simulink model "Assign_Task5and6"  (R2023a)
settings: Solver=ode1  StartTime=0.0  StopTime=30  FixedStep=Ts  MaxStep=Ts  RelTol=1e-3
model workspace (MAT data in the model file):
  wsw = 2000
values from neighbouring files (symbols this model uses):
  fg = 50    [Parameters.m]
  Rtpu = Xtpu/40    (= 0.00375)    [Parameters.m]
  S0non = 1000e6    (= 1000000000)    [Parameters.m]
  Svsc = 100e6    (= 100000000)    [Parameters.m]
  tonvsc = 1e-3    (= 0.001)    [Parameters.m]
  Ts = 20e-6    (= 2e-05)    [Parameters.m]
  Vhv = 22e3    (= 22000)    [Parameters.m]
  Vmv = 22e3    (= 22000)    [Parameters.m]
  wc1 = wsw1/10    (= 848.230016469)    [Parameters.m]
  wpq1 = wc1/10    (= 84.8230016469)    [Parameters.m]
  wsw1 = ksw1*2*pi*fg    (= 8482.30016469)    [Parameters.m]
  Xtpu = 0.15    [Parameters.m]
undefined symbols (not defined in the file or in its folder): D11, Delta, Kf, r, tfilt, theta0
libraries: simulink_extras x20, spsGroundLib x18, spsCurrentMeasurementLib x12, spsVoltageMeasurementLib x12, pid_lib x7, slpidlib x7, spsThreePhaseParallelRLCLoadLib x6, spsControlledVoltageSourceLib x6, powerlib_meascontrol x5, spsThreePhaseBreakerLib x4, eeTransforms x4, spsabctoAlphaBetaZeroLib x3
(part 3 of 3)

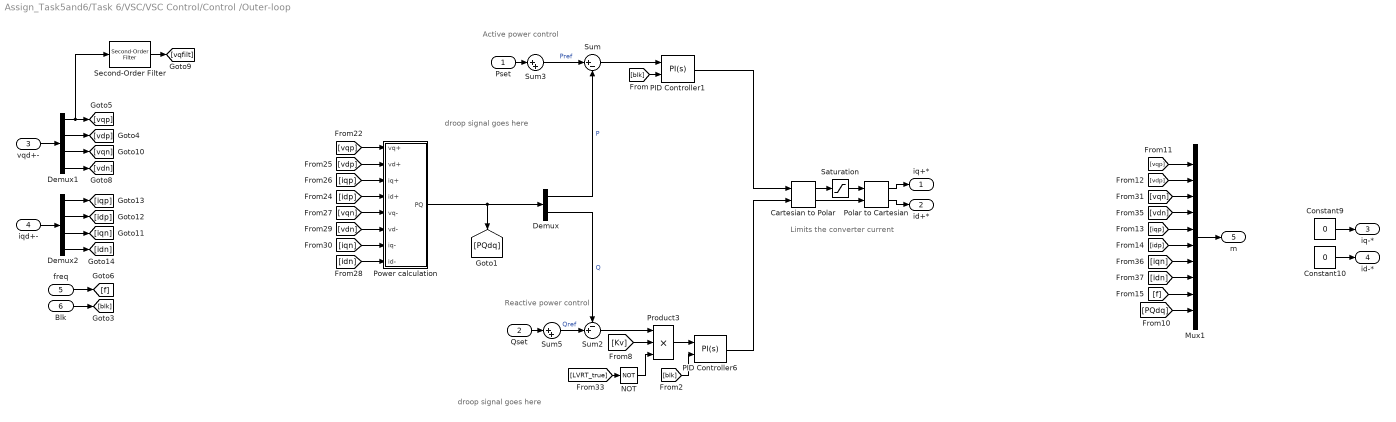
== system Assign_Task5and6/Task 6/VSC/VSC Control/Control /Outer-loop ==
  note: droop signal goes here
  note: Limits the converter current
  note: Reactive power control
  note: Active power control
  note: droop signal goes here
  Pset : Inport
  Qset : Inport  Port=2
  vqd+- : Inport  Port=3
  iqd+- : Inport  Port=4
  freq : Inport  Port=5
  Blk : Inport  Port=6
  Cartesian to Polar : simulink_extras/Transformations/Cartesian to Polar
  Constant10 : Constant  Value=0
  Constant9 : Constant  Value=0
  Demux : Demux  Outputs=2
  Demux1 : Demux
  Demux2 : Demux
  Mux1 : Mux  Inputs=10
  NOT : Logic  Operator=NOT  IconShape=distinctive  AllPortsSameDT=off  OutDataTypeStr=boolean
  PID Controller1 : slpidlib/PID Controller  Controller=PI  Form=Ideal  TimeDomain=Continuous-time  UseExternalTs=off  SampleTime=-1  IntegratorMethod=Forward Euler  FilterMethod=Forward Euler  ControllerParametersSource=internal  P=kp_pq  I=1/ti_pq  UseKiTs=off  D=0  N=100  UseFilter=on  TunerSelectOption=Transfer Function Based (PID Tuner App)  InitialConditionSource=internal  InitialConditionForIntegrator=0  InitialConditionForFilter=0  DifferentiatorICPrevScaledInput=0  ExternalReset=level  TrackingMode=off  Kt=1  LimitOutput=off  SatLimitsSource=internal  UpperSaturationLimit=inf  LowerSaturationLimit=-inf  LinearizeAsGain=on  AntiWindupMode=none  Kb=1  LimitIntegrator=off  UpperIntegratorSaturationLimit=inf  LowerIntegratorSaturationLimit=-inf  POutMin=[]  POutMax=[]  IOutMin=[]  IOutMax=[]  DOutMin=[]  DOutMax=[]  NOutMin=[]  NOutMax=[]  SumOutMin=[]  SumOutMax=[]  SaturationOutMin=[]  SaturationOutMax=[]  PParamMin=[]  PParamMax=[]  IParamMin=[]  IParamMax=[]  DParamMin=[]  DParamMax=[]  NParamMin=[]  NParamMax=[]  KbParamMin=[]  KbParamMax=[]  KtParamMin=[]  KtParamMax=[]  KbOutMin=[]  KbOutMax=[]  KtOutMin=[]  KtOutMax=[]  IntegratorOutMin=[]  IntegratorOutMax=[]  FilterOutMin=[]  FilterOutMax=[]  SumI1OutMin=[]  SumI1OutMax=[]  SumI2OutMin=[]  SumI2OutMax=[]  SumI3OutMin=[]  SumI3OutMax=[]  SumI4OutMin=[]  SumI4OutMax=[]  SumDOutMin=[]  SumDOutMax=[]  DifferentiatorOutMin=[]  DifferentiatorOutMax=[]  FilterDiffOutCoefMin=[]  FilterDiffOutCoefMax=[]  ReciprocalOutMin=[]  ReciprocalOutMax=[]  SumDenOutMin=[]  SumDenOutMax=[]  SumNumOutMin=[]  SumNumOutMax=[]  DivideOutMin=[]  DivideOutMax=[]  UdiffTsProdOutMin=[]  UdiffTsProdOutMax=[]  NTsProdOutMin=[]  NTsProdOutMax=[]  UintegralTsProdOutMin=[]  UintegralTsProdOutMax=[]  UngainTsProdOutMin=[]  UngainTsProdOutMax=[]  ClampingZeroOutDataTypeStr=Inherit: Inherit via back propagation  ClampingZeroOutMin=[]  ClampingZeroOutMax=[]  FilterDenConstantOutDataTypeStr=Inherit: Inherit via back propagation  FilterDenConstantOutMin=[]  FilterDenConstantOutMax=[]  PCopyOutDataTypeStr=Inherit: Inherit via back propagation  PCopyOutMin=[]  PCopyOutMax=[]  NCopyOutDataTypeStr=Inherit: Inherit via back propagation  NCopyOutMin=[]  NCopyOutMax=[]  IntegratorContinuousStateAttributes=''  IntegratorStateMustResolveToSignalObject=off  IntegratorRTWStateStorageClass=Auto  FilterContinuousStateAttributes=''  FilterStateMustResolveToSignalObject=off  FilterRTWStateStorageClass=Auto  ParallelPVariant=Passthrough  IdealPVariant=InternalParameters  IVariant=InternalParameters  DVariant=Disabled  IntegratorVariant=Continuous  SatVariant=Disabled  AWVariant=Passthrough  PCopyVariant=Disabled  TRVariant=Disabled  FdbkBlocksVariant=Forward  IdealPFdbkVariant=Disabled  SatFdbkVariant=Disabled  DerivativeFilterVariant=Disabled  NVariant=Disabled  NCopyVariant=Disabled_SignalSpec  FilterICVariant=Disabled  IntegratorICVariant=InternalICs  ExternalResetVariant=ExternalReset  TRSumVariant=Passthrough  SumFdbkVariant=Disabled  SumVariant=Sum_PI  TsampFilterVariant=InternalTs  TsampNgainVariant=Passthrough  TsampIntegralVariant=Disabled_SignalSpec  ExternalSaturationOutDataTypeStr=Inherit: Same as second input
  PID Controller6 : slpidlib/PID Controller  Controller=PI  Form=Ideal  TimeDomain=Continuous-time  UseExternalTs=off  SampleTime=-1  IntegratorMethod=Forward Euler  FilterMethod=Forward Euler  ControllerParametersSource=internal  P=kp_pq  I=1/ti_pq  UseKiTs=off  D=0  N=100  UseFilter=on  TunerSelectOption=Transfer Function Based (PID Tuner App)  InitialConditionSource=internal  InitialConditionForIntegrator=0  InitialConditionForFilter=0  DifferentiatorICPrevScaledInput=0  ExternalReset=level  TrackingMode=off  Kt=1  LimitOutput=off  SatLimitsSource=internal  UpperSaturationLimit=inf  LowerSaturationLimit=-inf  LinearizeAsGain=on  AntiWindupMode=none  Kb=1  LimitIntegrator=off  UpperIntegratorSaturationLimit=inf  LowerIntegratorSaturationLimit=-inf  POutMin=[]  POutMax=[]  IOutMin=[]  IOutMax=[]  DOutMin=[]  DOutMax=[]  NOutMin=[]  NOutMax=[]  SumOutMin=[]  SumOutMax=[]  SaturationOutMin=[]  SaturationOutMax=[]  PParamMin=[]  PParamMax=[]  IParamMin=[]  IParamMax=[]  DParamMin=[]  DParamMax=[]  NParamMin=[]  NParamMax=[]  KbParamMin=[]  KbParamMax=[]  KtParamMin=[]  KtParamMax=[]  KbOutMin=[]  KbOutMax=[]  KtOutMin=[]  KtOutMax=[]  IntegratorOutMin=[]  IntegratorOutMax=[]  FilterOutMin=[]  FilterOutMax=[]  SumI1OutMin=[]  SumI1OutMax=[]  SumI2OutMin=[]  SumI2OutMax=[]  SumI3OutMin=[]  SumI3OutMax=[]  SumI4OutMin=[]  SumI4OutMax=[]  SumDOutMin=[]  SumDOutMax=[]  DifferentiatorOutMin=[]  DifferentiatorOutMax=[]  FilterDiffOutCoefMin=[]  FilterDiffOutCoefMax=[]  ReciprocalOutMin=[]  ReciprocalOutMax=[]  SumDenOutMin=[]  SumDenOutMax=[]  SumNumOutMin=[]  SumNumOutMax=[]  DivideOutMin=[]  DivideOutMax=[]  UdiffTsProdOutMin=[]  UdiffTsProdOutMax=[]  NTsProdOutMin=[]  NTsProdOutMax=[]  UintegralTsProdOutMin=[]  UintegralTsProdOutMax=[]  UngainTsProdOutMin=[]  UngainTsProdOutMax=[]  ClampingZeroOutDataTypeStr=Inherit: Inherit via back propagation  ClampingZeroOutMin=[]  ClampingZeroOutMax=[]  FilterDenConstantOutDataTypeStr=Inherit: Inherit via back propagation  FilterDenConstantOutMin=[]  FilterDenConstantOutMax=[]  PCopyOutDataTypeStr=Inherit: Inherit via back propagation  PCopyOutMin=[]  PCopyOutMax=[]  NCopyOutDataTypeStr=Inherit: Inherit via back propagation  NCopyOutMin=[]  NCopyOutMax=[]  IntegratorContinuousStateAttributes=''  IntegratorStateMustResolveToSignalObject=off  IntegratorRTWStateStorageClass=Auto  FilterContinuousStateAttributes=''  FilterStateMustResolveToSignalObject=off  FilterRTWStateStorageClass=Auto  ParallelPVariant=Passthrough  IdealPVariant=InternalParameters  IVariant=InternalParameters  DVariant=Disabled  IntegratorVariant=Continuous  SatVariant=Disabled  AWVariant=Passthrough  PCopyVariant=Disabled  TRVariant=Disabled  FdbkBlocksVariant=Forward  IdealPFdbkVariant=Disabled  SatFdbkVariant=Disabled  DerivativeFilterVariant=Disabled  NVariant=Disabled  NCopyVariant=Disabled_SignalSpec  FilterICVariant=Disabled  IntegratorICVariant=InternalICs  ExternalResetVariant=ExternalReset  TRSumVariant=Passthrough  SumFdbkVariant=Disabled  SumVariant=Sum_PI  TsampFilterVariant=InternalTs  TsampNgainVariant=Passthrough  TsampIntegralVariant=Disabled_SignalSpec  ExternalSaturationOutDataTypeStr=Inherit: Same as second input
  Polar to Cartesian : simulink_extras/Transformations/Polar to Cartesian
  Power calculation : Subsystem
  Product3 : Product  Inputs=3
  Saturation : Saturate  UpperLimit=Imax  LowerLimit=0
  Second-Order Filter : eeGeneralControl/Second-Order Filter  FilterType=Low-pass  fn=150  Zeta=0.9  Ts=-1  A0=0  Ph0=0  f0=0  b0=0
  Sum : Sum  Inputs=|+-
  Sum2 : Sum  Inputs=-+|
  Sum3 : Sum  Inputs=|++
  Sum5 : Sum  Inputs=|++
  iq+* : Outport
  id+* : Outport  Port=2
  iq-* : Outport  Port=3
  id-* : Outport  Port=4
  m : Outport  Port=5
  wires:
  Constant10/1 -> id-*/1
  Constant9/1 -> iq-*/1
  Qset/1 -> Sum5/1
  Cartesian to Polar/2 -> Polar to Cartesian/2
  Polar to Cartesian/1 -> iq+*/1
  Polar to Cartesian/2 -> id+*/1
  Cartesian to Polar/1 -> Saturation/1
  Saturation/1 -> Polar to Cartesian/1
  Demux/1 -> Sum/2  "P"
  Demux/2 -> Sum2/1  "Q"
  Sum3/1 -> Sum/1  "Pref"
  Sum5/1 -> Sum2/2  "Qref"
  [Kv] -> Product3/2
  Sum2/1 -> Product3/1
  Pset/1 -> Sum3/1
  PID Controller1/1 -> Cartesian to Polar/1
  Blk/1 -> [blk]
  freq/1 -> [f]
  [vqp] -> Mux1/1
  Mux1/1 -> m/1
  Product3/1 -> PID Controller6/1
  Sum/1 -> PID Controller1/1
  Second-Order Filter/1 -> [vqfilt]
  vqd+-/1 -> Demux1/1
  iqd+-/1 -> Demux2/1
  Demux1/1 -> Second-Order Filter/1, [vqp]
  Demux1/2 -> [vdp]
  Demux1/3 -> [vqn]
  Demux1/4 -> [vdn]
  Demux2/1 -> [iqp]
  Demux2/2 -> [idp]
  Demux2/3 -> [iqn]
  Demux2/4 -> [idn]
  [vqp] -> Power calculation/1(vq+)
  [iqp] -> Power calculation/3(iq+)
  Power calculation/1(PQ) -> [PQdq], Demux/1
  [idp] -> Power calculation/4(id+)
  [vdp] -> Power calculation/2(vd+)
  [vqn] -> Power calculation/5(vq-)
  [vdn] -> Power calculation/6(vd-)
  [iqn] -> Power calculation/7(iq-)
  [idn] -> Power calculation/8(id-)
  [LVRT_true] -> NOT/1
  NOT/1 -> Product3/3
  PID Controller6/1 -> Cartesian to Polar/2
  [vdp] -> Mux1/2
  [vqn] -> Mux1/3
  [vdn] -> Mux1/4
  [iqn] -> Mux1/7
  [idn] -> Mux1/8
  [f] -> Mux1/9
  [PQdq] -> Mux1/10
  [idp] -> Mux1/6
  [iqp] -> Mux1/5
  [blk] -> PID Controller1/2
  [blk] -> PID Controller6/2
  ? -> Sum5/2
  ? -> Sum3/2

== system Assign_Task5and6/Task 6/VSC/VSC Control/Measurement and PLL/PLL aligned with positive-sequence ==
  note: PLL
      | aligned with vd+
  Vabc : Inport
  0-vd=-vd : Gain  Gain=-1
  Clock : Clock  Commented=on
  Constant : Constant  Commented=on  Value=2*pi*fg
  Constant1 : Constant  Commented=on  Value=2*pi
  Constant2 : Constant  Commented=on  Value=2*pi
  Filter : Constant  Commented=on  Value=-tfilt*fg*2*pi
  Gain : Gain  Gain=1/(2*pi)
  Integrator : Integrator
  Mod : Math  Commented=on  Operator=mod
  Mod1 : Math  Commented=on  Operator=mod
  Notch filter : Subsystem  Commented=through
  PID Controller : slpidlib/PID Controller  Commented=on  Controller=PI  Form=Ideal  TimeDomain=Continuous-time  UseExternalTs=off  SampleTime=-1  IntegratorMethod=Forward Euler  FilterMethod=Forward Euler  ControllerParametersSource=internal  P=kp_pll  I=1/tau_pll  UseKiTs=off  D=0  N=100  UseFilter=on  TunerSelectOption=Transfer Function Based (PID Tuner App)  InitialConditionSource=internal  InitialConditionForIntegrator=2*pi*fg  InitialConditionForFilter=0  DifferentiatorICPrevScaledInput=0  ExternalReset=none  TrackingMode=off  Kt=1  LimitOutput=off  SatLimitsSource=internal  UpperSaturationLimit=1.1*2*pi*fg  LowerSaturationLimit=0.9*2*pi*fg  LinearizeAsGain=on  AntiWindupMode=clamping  Kb=1/kp_pll  LimitIntegrator=off  UpperIntegratorSaturationLimit=inf  LowerIntegratorSaturationLimit=-inf  POutMin=[]  POutMax=[]  IOutMin=[]  IOutMax=[]  DOutMin=[]  DOutMax=[]  NOutMin=[]  NOutMax=[]  SumOutMin=[]  SumOutMax=[]  SaturationOutMin=[]  SaturationOutMax=[]  PParamMin=[]  PParamMax=[]  IParamMin=[]  IParamMax=[]  DParamMin=[]  DParamMax=[]  NParamMin=[]  NParamMax=[]  KbParamMin=[]  KbParamMax=[]  KtParamMin=[]  KtParamMax=[]  KbOutMin=[]  KbOutMax=[]  KtOutMin=[]  KtOutMax=[]  IntegratorOutMin=[]  IntegratorOutMax=[]  FilterOutMin=[]  FilterOutMax=[]  SumI1OutMin=[]  SumI1OutMax=[]  SumI2OutMin=[]  SumI2OutMax=[]  SumI3OutMin=[]  SumI3OutMax=[]  SumI4OutMin=[]  SumI4OutMax=[]  SumDOutMin=[]  SumDOutMax=[]  DifferentiatorOutMin=[]  DifferentiatorOutMax=[]  FilterDiffOutCoefMin=[]  FilterDiffOutCoefMax=[]  ReciprocalOutMin=[]  ReciprocalOutMax=[]  SumDenOutMin=[]  SumDenOutMax=[]  SumNumOutMin=[]  SumNumOutMax=[]  DivideOutMin=[]  DivideOutMax=[]  UdiffTsProdOutMin=[]  UdiffTsProdOutMax=[]  NTsProdOutMin=[]  NTsProdOutMax=[]  UintegralTsProdOutMin=[]  UintegralTsProdOutMax=[]  UngainTsProdOutMin=[]  UngainTsProdOutMax=[]  ClampingZeroOutDataTypeStr=Inherit: Inherit via back propagation  ClampingZeroOutMin=[]  ClampingZeroOutMax=[]  FilterDenConstantOutDataTypeStr=Inherit: Inherit via back propagation  FilterDenConstantOutMin=[]  FilterDenConstantOutMax=[]  PCopyOutDataTypeStr=Inherit: Inherit via back propagation  PCopyOutMin=[]  PCopyOutMax=[]  NCopyOutDataTypeStr=Inherit: Inherit via back propagation  NCopyOutMin=[]  NCopyOutMax=[]  IntegratorContinuousStateAttributes=''  IntegratorStateMustResolveToSignalObject=off  IntegratorRTWStateStorageClass=Auto  FilterContinuousStateAttributes=''  FilterStateMustResolveToSignalObject=off  FilterRTWStateStorageClass=Auto  ParallelPVariant=Passthrough  IdealPVariant=InternalParameters  IVariant=InternalParameters  DVariant=Disabled  IntegratorVariant=Continuous  SatVariant=Disabled  AWVariant=Passthrough  PCopyVariant=Disabled  TRVariant=Disabled  FdbkBlocksVariant=Forward  IdealPFdbkVariant=Disabled  SatFdbkVariant=Disabled  DerivativeFilterVariant=Disabled  NVariant=Disabled  NCopyVariant=Disabled_SignalSpec  FilterICVariant=Disabled  IntegratorICVariant=InternalICs  ExternalResetVariant=Disabled  TRSumVariant=Passthrough  SumFdbkVariant=Disabled  SumVariant=Sum_PI  TsampFilterVariant=InternalTs  TsampNgainVariant=Passthrough  TsampIntegralVariant=Disabled_SignalSpec  ExternalSaturationOutDataTypeStr=Inherit: Same as second input
  Park transform : Subsystem  Commented=on
  Phase-sequence separation : Subsystem
  Subsystem : Subsystem
      mask Display: disp('PI\n')
  Switch : Switch  Commented=on  Criteria=u2 > Threshold  Threshold=0.3  SaturateOnIntegerOverflow=off  InputSameDT=off
  Terminator : Terminator
  Terminator1 : Terminator
  Terminator2 : Terminator
  Transformer Y/D1 : Constant  Commented=on  Value=-pi/6
  theta : Outport
  f : Outport  Port=2
  wires:
  Integrator/1 -> theta/1, Phase-sequence separation/2(Theta)
  Constant2/1 -> Mod1/1
  Constant1/1 -> Mod/2
  Gain/1 -> f/1
  0-vd=-vd/1 -> Subsystem/1(in)
  Clock/1 -> Switch/2
  Constant/1 -> Switch/1
  Subsystem/1(w) -> Gain/1, Integrator/1
  Vabc/1 -> Phase-sequence separation/1(abc)
  Phase-sequence separation/1(q+) -> Terminator/1
  Phase-sequence separation/2(d+) -> 0-vd=-vd/1  "vd+"
  Phase-sequence separation/3(q-) -> Terminator1/1
  Phase-sequence separation/4(d-) -> Terminator2/1

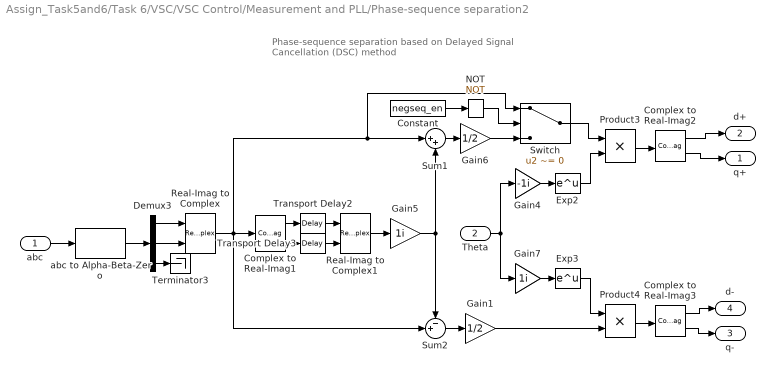
== system Assign_Task5and6/Task 6/VSC/VSC Control/Measurement and PLL/Phase-sequence separation2 ==
  note: Phase-sequence separation based on
      | Delayed Signal Cancellation (DSC) method
  abc : Inport
  Theta : Inport  Port=2
  Complex to Real-Imag1 : ComplexToRealImag
  Complex to Real-Imag2 : ComplexToRealImag
  Complex to Real-Imag3 : ComplexToRealImag
  Constant : Constant  Value=negseq_en
  Demux3 : Demux  Outputs=3
  Exp2 : Math  OutputSignalType=complex
  Exp3 : Math  OutputSignalType=complex
  Gain1 : Gain  Gain=1/2
  Gain4 : Gain  Gain=-1i
  Gain5 : Gain  Gain=1i
  Gain6 : Gain  Gain=1/2
  Gain7 : Gain  Gain=1i
  NOT : Logic  Operator=NOT  IconShape=distinctive  AllPortsSameDT=off  OutDataTypeStr=boolean
  Product3 : Product
  Product4 : Product
  Real-Imag to Complex : RealImagToComplex
  Real-Imag to Complex1 : RealImagToComplex
  Sum1 : Sum  Inputs=|++
  Sum2 : Sum  Inputs=-+|
  Switch : Switch  Criteria=u2 ~= 0  SaturateOnIntegerOverflow=off  InputSameDT=off
  Terminator3 : Terminator
  Transport Delay2 : TransportDelay  DelayTime=1/4*(1/50)
  Transport Delay3 : TransportDelay  DelayTime=1/4*(1/50)
  abc to Alpha-Beta-Zero : spsabctoAlphaBetaZeroLib/abc to Alpha-Beta-Zero
  q+ : Outport
  d+ : Outport  Port=2
  q- : Outport  Port=3
  d- : Outport  Port=4
  wires:
  NOT/1 -> Switch/2
  Constant/1 -> NOT/1
  Switch/1 -> Product3/1
  Gain6/1 -> Switch/3
  Sum2/1 -> Gain1/1
  Transport Delay2/1 -> Real-Imag to Complex1/1
  Demux3/1 -> Real-Imag to Complex/1
  Complex to Real-Imag1/2 -> Transport Delay3/1
  Gain1/1 -> Product4/2
  Real-Imag to Complex/1 -> Complex to Real-Imag1/1, Sum2/2, Sum1/1, Switch/1
  Complex to Real-Imag3/1 -> d-/1
  Real-Imag to Complex1/1 -> Gain5/1
  Complex to Real-Imag1/1 -> Transport Delay2/1
  Transport Delay3/1 -> Real-Imag to Complex1/2
  Demux3/2 -> Real-Imag to Complex/2
  Product3/1 -> Complex to Real-Imag2/1
  Product4/1 -> Complex to Real-Imag3/1
  abc to Alpha-Beta-Zero/1 -> Demux3/1
  abc/1 -> abc to Alpha-Beta-Zero/1
  Exp3/1 -> Product4/1
  Complex to Real-Imag3/2 -> q-/1
  Complex to Real-Imag2/2 -> q+/1
  Demux3/3 -> Terminator3/1
  Sum1/1 -> Gain6/1
  Gain5/1 -> Sum2/1, Sum1/2
  Exp2/1 -> Product3/2
  Gain4/1 -> Exp2/1
  Theta/1 -> Gain4/1, Gain7/1
  Gain7/1 -> Exp3/1
  Complex to Real-Imag2/1 -> d+/1

== system Assign_Task5and6/Task 6/VSC/VSC Control/Measurement and PLL/Phase-sequence separation3 ==
  note: Phase-sequence separation based on
      | Delayed Signal Cancellation (DSC) method
  abc : Inport
  Theta : Inport  Port=2
  Complex to Real-Imag1 : ComplexToRealImag
  Complex to Real-Imag2 : ComplexToRealImag
  Complex to Real-Imag3 : ComplexToRealImag
  Constant : Constant  Value=negseq_en
  Demux3 : Demux  Outputs=3
  Exp2 : Math  OutputSignalType=complex
  Exp3 : Math  OutputSignalType=complex
  Gain1 : Gain  Gain=1/2
  Gain4 : Gain  Gain=-1i
  Gain5 : Gain  Gain=1i
  Gain6 : Gain  Gain=1/2
  Gain7 : Gain  Gain=1i
  NOT : Logic  Operator=NOT  IconShape=distinctive  AllPortsSameDT=off  OutDataTypeStr=boolean
  Product3 : Product
  Product4 : Product
  Real-Imag to Complex : RealImagToComplex
  Real-Imag to Complex1 : RealImagToComplex
  Sum1 : Sum  Inputs=|++
  Sum2 : Sum  Inputs=-+|
  Switch : Switch  Criteria=u2 ~= 0  SaturateOnIntegerOverflow=off  InputSameDT=off
  Terminator3 : Terminator
  Transport Delay2 : TransportDelay  DelayTime=1/4*(1/50)
  Transport Delay3 : TransportDelay  DelayTime=1/4*(1/50)
  abc to Alpha-Beta-Zero : spsabctoAlphaBetaZeroLib/abc to Alpha-Beta-Zero
  q+ : Outport
  d+ : Outport  Port=2
  q- : Outport  Port=3
  d- : Outport  Port=4
  wires:
  Complex to Real-Imag2/1 -> d+/1
  Gain7/1 -> Exp3/1
  Theta/1 -> Gain7/1, Gain4/1
  Gain4/1 -> Exp2/1
  Exp2/1 -> Product3/2
  Gain5/1 -> Sum1/2, Sum2/1
  Sum1/1 -> Gain6/1
  Demux3/3 -> Terminator3/1
  Complex to Real-Imag2/2 -> q+/1
  Complex to Real-Imag3/2 -> q-/1
  Exp3/1 -> Product4/1
  abc/1 -> abc to Alpha-Beta-Zero/1
  abc to Alpha-Beta-Zero/1 -> Demux3/1
  Product4/1 -> Complex to Real-Imag3/1
  Product3/1 -> Complex to Real-Imag2/1
  Demux3/2 -> Real-Imag to Complex/2
  Transport Delay3/1 -> Real-Imag to Complex1/2
  Complex to Real-Imag1/1 -> Transport Delay2/1
  Real-Imag to Complex1/1 -> Gain5/1
  Complex to Real-Imag3/1 -> d-/1
  Real-Imag to Complex/1 -> Switch/1, Sum1/1, Sum2/2, Complex to Real-Imag1/1
  Gain1/1 -> Product4/2
  Complex to Real-Imag1/2 -> Transport Delay3/1
  Demux3/1 -> Real-Imag to Complex/1
  Transport Delay2/1 -> Real-Imag to Complex1/1
  Sum2/1 -> Gain1/1
  Gain6/1 -> Switch/3
  Switch/1 -> Product3/1
  Constant/1 -> NOT/1
  NOT/1 -> Switch/2

== system Assign_Task5and6/Task 6/VSC/VSC Control/Modulation/Corrects delay ==
  Clock : Clock
  Filter delay : Constant  Commented=on  Value=tfilt
  Gain : Gain  Gain=2*pi*fg
  Memory : Memory
  Sum : Sum  Inputs=|+-
  Sum1 : Sum  Inputs=|++
  Sum2 : Sum  Inputs=|++
  Transformer connection : Constant  Value=pi/6
  dphi : Outport
  wires:
  Clock/1 -> Memory/1, Sum/1
  Memory/1 -> Sum/2
  Sum1/1 -> Gain/1  "Td"
  Sum/1 -> Sum1/1  "Ts"
  Filter delay/1 -> Sum1/2  "Tf"
  Gain/1 -> Sum2/1
  Sum2/1 -> dphi/1
  Transformer connection/1 -> Sum2/2  "Tf"

== system Assign_Task5and6/Task 6/VSC/VSC Control/Modulation/Corrects delay1 ==
  Clock : Clock
  Filter delay : Constant  Commented=on  Value=tfilt
  Gain : Gain  Gain=-2*pi*fg
  Gain1 : Gain
  Memory : Memory
  Sum : Sum  Inputs=|+-
  Sum1 : Sum  Inputs=|++
  Sum2 : Sum  Inputs=|++
  Transformer connection : Constant  Value=pi/6
  dphi : Outport
  wires:
  Clock/1 -> Memory/1, Sum/1
  Memory/1 -> Sum/2
  Sum1/1 -> Gain/1  "Td"
  Sum/1 -> Sum1/1  "Ts"
  Filter delay/1 -> Sum1/2  "Tf"
  Gain/1 -> Sum2/1
  Sum2/1 -> Gain1/1
  Transformer connection/1 -> Sum2/2  "Tf"
  Gain1/1 -> dphi/1

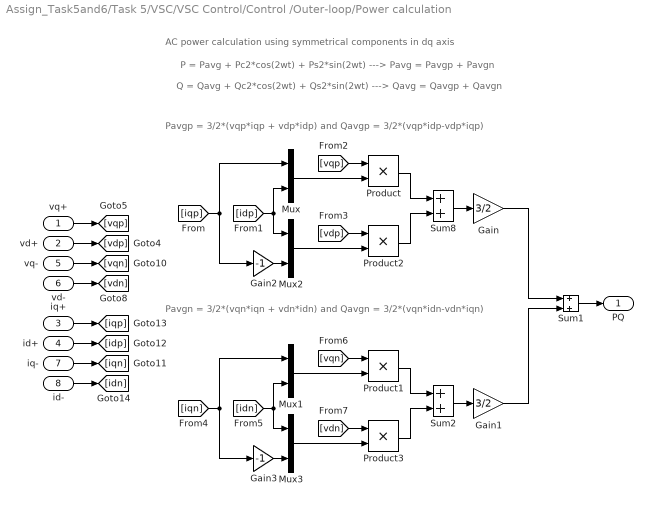
== system Assign_Task5and6/Task 5/VSC/VSC Control/Control /Outer-loop/Power calculation ==
  note: AC power calculation using symmetrical components in dq axis
  note: Pavgp = 3/2*(vqp*iqp + vdp*idp) and Qavgp = 3/2*(vqp*idp-vdp*iqp)
  note: P = Pavg + Pc2*cos(2wt) + Ps2*sin(2wt) ---> Pavg = Pavgp + Pavgn
  note: Q = Qavg + Qc2*cos(2wt) + Qs2*sin(2wt) ---> Qavg = Qavgp + Qavgn
  note: Pavgn = 3/2*(vqn*iqn + vdn*idn) and Qavgn = 3/2*(vqn*idn-vdn*iqn)
  vq+ : Inport
  vd+ : Inport  Port=2
  iq+ : Inport  Port=3
  id+ : Inport  Port=4
  vq- : Inport  Port=5
  vd- : Inport  Port=6
  iq- : Inport  Port=7
  id- : Inport  Port=8
  Gain : Gain  Gain=3/2
  Gain1 : Gain  Gain=3/2
  Gain2 : Gain  Gain=-1
  Gain3 : Gain  Gain=-1
  Mux{,1..3} (4 alike) : Mux  Inputs=2
  Product{,1..3} (4 alike) : Product
  Sum1 : Sum
  Sum2 : Sum
  Sum8 : Sum
  PQ : Outport
  wires:
  Sum8/1 -> Gain/1
  Gain2/1 -> Mux2/2
  Mux2/1 -> Product2/2
  Product2/1 -> Sum8/2
  Mux/1 -> Product/2
  Product/1 -> Sum8/1
  iq+/1 -> [iqp]
  [iqp] -> Gain2/1, Mux/1
  id+/1 -> [idp]
  [idp] -> Mux2/1, Mux/2
  vq+/1 -> [vqp]
  [vqp] -> Product/1
  vd+/1 -> [vdp]
  [vdp] -> Product2/1
  Gain/1 -> Sum1/1
  Sum1/1 -> PQ/1
  Gain3/1 -> Mux3/2
  Mux1/1 -> Product1/2
  Product3/1 -> Sum2/2
  Product1/1 -> Sum2/1
  [vdn] -> Product3/1
  Mux3/1 -> Product3/2
  [vqn] -> Product1/1
  Sum2/1 -> Gain1/1
  [iqn] -> Gain3/1, Mux1/1
  [idn] -> Mux3/1, Mux1/2
  vq-/1 -> [vqn]
  vd-/1 -> [vdn]
  iq-/1 -> [iqn]
  id-/1 -> [idn]
  Gain1/1 -> Sum1/2

== system Assign_Task5and6/Task 5/VSC/VSC Control/Measurement and PLL/PLL aligned with positive-sequence/Notch filter ==
  In : Inport
  Discrete Transfer Fcn : DiscreteTransferFcn  Numerator=[1, -2*cos(theta0), 1]  Denominator="[1, -2*cos(theta0)*r,  r^2]"
  Gain7 : Gain  Gain=Kf
  Out : Outport
  wires:
  Gain7/1 -> Discrete Transfer Fcn/1
  Discrete Transfer Fcn/1 -> Out/1
  In/1 -> Gain7/1

== system Assign_Task5and6/Task 5/VSC/VSC Control/Measurement and PLL/PLL aligned with positive-sequence/Park transform ==
  note: Park transform (q axis leading)
  abc : Inport
  theta : Inport  Port=2
  0 : Fcn  Expr=1/3*(u(1) + u(2) + u(3))
  Mux2 : Mux  Inputs=2
  Mux3 : Mux  Inputs=3
  d : Fcn  Expr=2/3*(u(1)*sin(u(4)) + u(2)*sin(u(4) - (2*pi)/3) + u(3)*sin(u(4) + (2*pi)/3))
  q : Fcn  Expr=2/3*(u(1)*cos(u(4)) + u(2)*cos(u(4) - (2*pi)/3) + u(3)*cos(u(4) + (2*pi)/3))
  qd0 : Outport  VectorParamsAs1DForOutWhenUnconnected=off
  wires:
  q/1 -> Mux3/1
  Mux2/1 -> q/1, 0/1, d/1
  0/1 -> Mux3/3
  d/1 -> Mux3/2
  theta/1 -> Mux2/2
  abc/1 -> Mux2/1
  Mux3/1 -> qd0/1

== system Assign_Task5and6/Task 5/VSC/VSC Control/Measurement and PLL/PLL aligned with positive-sequence/Phase-sequence separation ==
  note: Phase-sequence separation based on
      | Delayed Signal Cancellation (DSC) method
  abc : Inport
  Theta : Inport  Port=2
  Complex to Real-Imag1 : ComplexToRealImag
  Complex to Real-Imag2 : ComplexToRealImag
  Complex to Real-Imag3 : ComplexToRealImag
  Constant : Constant  Value=negseq_en
  Demux3 : Demux  Outputs=3
  Exp2 : Math  OutputSignalType=complex
  Exp3 : Math  OutputSignalType=complex
  Gain1 : Gain  Gain=1/2
  Gain4 : Gain  Gain=-1i
  Gain5 : Gain  Gain=1i
  Gain6 : Gain  Gain=1/2
  Gain7 : Gain  Gain=1i
  NOT : Logic  Operator=NOT  IconShape=distinctive  AllPortsSameDT=off  OutDataTypeStr=boolean
  Product3 : Product
  Product4 : Product
  Real-Imag to Complex : RealImagToComplex
  Real-Imag to Complex1 : RealImagToComplex
  Sum1 : Sum  Inputs=|++
  Sum2 : Sum  Inputs=-+|
  Switch : Switch  Criteria=u2 ~= 0  SaturateOnIntegerOverflow=off  InputSameDT=off
  Terminator3 : Terminator
  Transport Delay2 : TransportDelay  DelayTime=1/4*(1/50)
  Transport Delay3 : TransportDelay  DelayTime=1/4*(1/50)
  abc to Alpha-Beta-Zero : powerlib_meascontrol/Transformations/abc to Alpha-Beta-Zero
  q+ : Outport
  d+ : Outport  Port=2
  q- : Outport  Port=3
  d- : Outport  Port=4
  wires:
  NOT/1 -> Switch/2
  Constant/1 -> NOT/1
  Switch/1 -> Product3/1
  Gain6/1 -> Switch/3
  Sum2/1 -> Gain1/1
  Transport Delay2/1 -> Real-Imag to Complex1/1
  Demux3/1 -> Real-Imag to Complex/1
  Complex to Real-Imag1/2 -> Transport Delay3/1
  Gain1/1 -> Product4/2
  Real-Imag to Complex/1 -> Complex to Real-Imag1/1, Sum2/2, Sum1/1, Switch/1
  Complex to Real-Imag3/1 -> d-/1
  Real-Imag to Complex1/1 -> Gain5/1
  Complex to Real-Imag1/1 -> Transport Delay2/1
  Transport Delay3/1 -> Real-Imag to Complex1/2
  Demux3/2 -> Real-Imag to Complex/2
  Product3/1 -> Complex to Real-Imag2/1
  Product4/1 -> Complex to Real-Imag3/1
  abc to Alpha-Beta-Zero/1 -> Demux3/1
  abc/1 -> abc to Alpha-Beta-Zero/1
  Exp3/1 -> Product4/1
  Complex to Real-Imag3/2 -> q-/1
  Complex to Real-Imag2/2 -> q+/1
  Demux3/3 -> Terminator3/1
  Sum1/1 -> Gain6/1
  Gain5/1 -> Sum2/1, Sum1/2
  Exp2/1 -> Product3/2
  Gain4/1 -> Exp2/1
  Theta/1 -> Gain4/1, Gain7/1
  Gain7/1 -> Exp3/1
  Complex to Real-Imag2/1 -> d+/1

== system Assign_Task5and6/Task 5/VSC/VSC Control/Measurement and PLL/PLL aligned with positive-sequence/Subsystem ==
  note: PI controller with reset port and initial conditions restored after reset or after maximum/minimum values are reached
  in : Inport
  Reset : Inport  Port=2
  Compare To Constant2 : simulink/Logic and Bit Operations/Compare To Constant  relop=~=  const=0  OutDataTypeStr=boolean
  Constant2 : Constant  Value=2*pi*fg
  Gain : Gain  Gain=kp_pll
  Gain1 : Gain  Gain=kp_pll/tau_pll
  Integrator Limited : Integrator  ExternalReset=level  InitialCondition=2*pi*fg  UpperSaturationLimit=10.1*2*pi*fg  LowerSaturationLimit=0.09*2*pi*fg  ShowSaturationPort=on
  Memory1 : Memory
  NOT : Logic  Operator=NOT  IconShape=distinctive  AllPortsSameDT=off  OutDataTypeStr=boolean
  OR2 : Logic  Operator=OR  IconShape=distinctive  AllPortsSameDT=off  OutDataTypeStr=boolean
  Product : Product
  Sum : Sum
  Switch1 : Switch  SaturateOnIntegerOverflow=off  InputSameDT=off
  w : Outport
  wires:
  Switch1/1 -> w/1
  Product/1 -> Gain1/1, Gain/1
  Gain1/1 -> Integrator Limited/1
  Integrator Limited/2 -> Compare To Constant2/1, Switch1/2
  Compare To Constant2/1 -> Memory1/1
  OR2/1 -> Integrator Limited/2, NOT/1
  Constant2/1 -> Switch1/3
  Memory1/1 -> OR2/1
  Reset/1 -> OR2/2
  Gain/1 -> Sum/1
  Integrator Limited/1 -> Sum/2
  Sum/1 -> Switch1/1
  in/1 -> Product/1
  NOT/1 -> Product/2

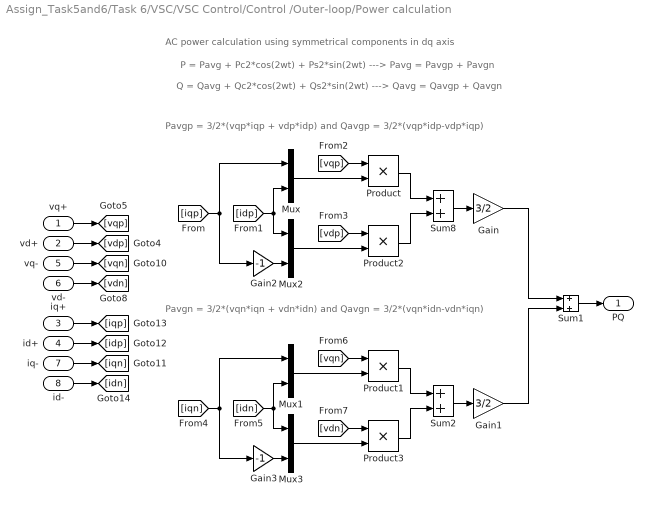
== system Assign_Task5and6/Task 6/VSC/VSC Control/Control /Outer-loop/Power calculation ==
  note: AC power calculation using symmetrical components in dq axis
  note: Pavgp = 3/2*(vqp*iqp + vdp*idp) and Qavgp = 3/2*(vqp*idp-vdp*iqp)
  note: P = Pavg + Pc2*cos(2wt) + Ps2*sin(2wt) ---> Pavg = Pavgp + Pavgn
  note: Q = Qavg + Qc2*cos(2wt) + Qs2*sin(2wt) ---> Qavg = Qavgp + Qavgn
  note: Pavgn = 3/2*(vqn*iqn + vdn*idn) and Qavgn = 3/2*(vqn*idn-vdn*iqn)
  vq+ : Inport
  vd+ : Inport  Port=2
  iq+ : Inport  Port=3
  id+ : Inport  Port=4
  vq- : Inport  Port=5
  vd- : Inport  Port=6
  iq- : Inport  Port=7
  id- : Inport  Port=8
  Gain : Gain  Gain=3/2
  Gain1 : Gain  Gain=3/2
  Gain2 : Gain  Gain=-1
  Gain3 : Gain  Gain=-1
  Mux{,1..3} (4 alike) : Mux  Inputs=2
  Product{,1..3} (4 alike) : Product
  Sum1 : Sum
  Sum2 : Sum
  Sum8 : Sum
  PQ : Outport
  wires:
  Sum8/1 -> Gain/1
  Gain2/1 -> Mux2/2
  Mux2/1 -> Product2/2
  Product2/1 -> Sum8/2
  Mux/1 -> Product/2
  Product/1 -> Sum8/1
  iq+/1 -> [iqp]
  [iqp] -> Gain2/1, Mux/1
  id+/1 -> [idp]
  [idp] -> Mux2/1, Mux/2
  vq+/1 -> [vqp]
  [vqp] -> Product/1
  vd+/1 -> [vdp]
  [vdp] -> Product2/1
  Gain/1 -> Sum1/1
  Sum1/1 -> PQ/1
  Gain3/1 -> Mux3/2
  Mux1/1 -> Product1/2
  Product3/1 -> Sum2/2
  Product1/1 -> Sum2/1
  [vdn] -> Product3/1
  Mux3/1 -> Product3/2
  [vqn] -> Product1/1
  Sum2/1 -> Gain1/1
  [iqn] -> Gain3/1, Mux1/1
  [idn] -> Mux3/1, Mux1/2
  vq-/1 -> [vqn]
  vd-/1 -> [vdn]
  iq-/1 -> [iqn]
  id-/1 -> [idn]
  Gain1/1 -> Sum1/2

== system Assign_Task5and6/Task 6/VSC/VSC Control/Measurement and PLL/PLL aligned with positive-sequence/Notch filter ==
  In : Inport
  Discrete Transfer Fcn : DiscreteTransferFcn  Numerator=[1, -2*cos(theta0), 1]  Denominator="[1, -2*cos(theta0)*r,  r^2]"
  Gain7 : Gain  Gain=Kf
  Out : Outport
  wires:
  Gain7/1 -> Discrete Transfer Fcn/1
  Discrete Transfer Fcn/1 -> Out/1
  In/1 -> Gain7/1

== system Assign_Task5and6/Task 6/VSC/VSC Control/Measurement and PLL/PLL aligned with positive-sequence/Park transform ==
  note: Park transform (q axis leading)
  abc : Inport
  theta : Inport  Port=2
  0 : Fcn  Expr=1/3*(u(1) + u(2) + u(3))
  Mux2 : Mux  Inputs=2
  Mux3 : Mux  Inputs=3
  d : Fcn  Expr=2/3*(u(1)*sin(u(4)) + u(2)*sin(u(4) - (2*pi)/3) + u(3)*sin(u(4) + (2*pi)/3))
  q : Fcn  Expr=2/3*(u(1)*cos(u(4)) + u(2)*cos(u(4) - (2*pi)/3) + u(3)*cos(u(4) + (2*pi)/3))
  qd0 : Outport  VectorParamsAs1DForOutWhenUnconnected=off
  wires:
  q/1 -> Mux3/1
  Mux2/1 -> q/1, 0/1, d/1
  0/1 -> Mux3/3
  d/1 -> Mux3/2
  theta/1 -> Mux2/2
  abc/1 -> Mux2/1
  Mux3/1 -> qd0/1

== system Assign_Task5and6/Task 6/VSC/VSC Control/Measurement and PLL/PLL aligned with positive-sequence/Phase-sequence separation ==
  note: Phase-sequence separation based on
      | Delayed Signal Cancellation (DSC) method
  abc : Inport
  Theta : Inport  Port=2
  Complex to Real-Imag1 : ComplexToRealImag
  Complex to Real-Imag2 : ComplexToRealImag
  Complex to Real-Imag3 : ComplexToRealImag
  Constant : Constant  Value=negseq_en
  Demux3 : Demux  Outputs=3
  Exp2 : Math  OutputSignalType=complex
  Exp3 : Math  OutputSignalType=complex
  Gain1 : Gain  Gain=1/2
  Gain4 : Gain  Gain=-1i
  Gain5 : Gain  Gain=1i
  Gain6 : Gain  Gain=1/2
  Gain7 : Gain  Gain=1i
  NOT : Logic  Operator=NOT  IconShape=distinctive  AllPortsSameDT=off  OutDataTypeStr=boolean
  Product3 : Product
  Product4 : Product
  Real-Imag to Complex : RealImagToComplex
  Real-Imag to Complex1 : RealImagToComplex
  Sum1 : Sum  Inputs=|++
  Sum2 : Sum  Inputs=-+|
  Switch : Switch  Criteria=u2 ~= 0  SaturateOnIntegerOverflow=off  InputSameDT=off
  Terminator3 : Terminator
  Transport Delay2 : TransportDelay  DelayTime=1/4*(1/50)
  Transport Delay3 : TransportDelay  DelayTime=1/4*(1/50)
  abc to Alpha-Beta-Zero : spsabctoAlphaBetaZeroLib/abc to Alpha-Beta-Zero
  q+ : Outport
  d+ : Outport  Port=2
  q- : Outport  Port=3
  d- : Outport  Port=4
  wires:
  NOT/1 -> Switch/2
  Constant/1 -> NOT/1
  Switch/1 -> Product3/1
  Gain6/1 -> Switch/3
  Sum2/1 -> Gain1/1
  Transport Delay2/1 -> Real-Imag to Complex1/1
  Demux3/1 -> Real-Imag to Complex/1
  Complex to Real-Imag1/2 -> Transport Delay3/1
  Gain1/1 -> Product4/2
  Real-Imag to Complex/1 -> Complex to Real-Imag1/1, Sum2/2, Sum1/1, Switch/1
  Complex to Real-Imag3/1 -> d-/1
  Real-Imag to Complex1/1 -> Gain5/1
  Complex to Real-Imag1/1 -> Transport Delay2/1
  Transport Delay3/1 -> Real-Imag to Complex1/2
  Demux3/2 -> Real-Imag to Complex/2
  Product3/1 -> Complex to Real-Imag2/1
  Product4/1 -> Complex to Real-Imag3/1
  abc to Alpha-Beta-Zero/1 -> Demux3/1
  abc/1 -> abc to Alpha-Beta-Zero/1
  Exp3/1 -> Product4/1
  Complex to Real-Imag3/2 -> q-/1
  Complex to Real-Imag2/2 -> q+/1
  Demux3/3 -> Terminator3/1
  Sum1/1 -> Gain6/1
  Gain5/1 -> Sum2/1, Sum1/2
  Exp2/1 -> Product3/2
  Gain4/1 -> Exp2/1
  Theta/1 -> Gain4/1, Gain7/1
  Gain7/1 -> Exp3/1
  Complex to Real-Imag2/1 -> d+/1

== system Assign_Task5and6/Task 6/VSC/VSC Control/Measurement and PLL/PLL aligned with positive-sequence/Subsystem ==
  note: PI controller with reset port and initial conditions restored after reset or after maximum/minimum values are reached
  in : Inport
  Reset : Inport  Port=2
  Compare To Constant2 : simulink/Logic and Bit Operations/Compare To Constant  relop=~=  const=0  OutDataTypeStr=boolean
  Constant2 : Constant  Value=2*pi*fg
  Gain : Gain  Gain=kp_pll
  Gain1 : Gain  Gain=kp_pll/tau_pll
  Integrator Limited : Integrator  ExternalReset=level  InitialCondition=2*pi*fg  UpperSaturationLimit=10.1*2*pi*fg  LowerSaturationLimit=0.09*2*pi*fg  ShowSaturationPort=on
  Memory1 : Memory
  NOT : Logic  Operator=NOT  IconShape=distinctive  AllPortsSameDT=off  OutDataTypeStr=boolean
  OR2 : Logic  Operator=OR  IconShape=distinctive  AllPortsSameDT=off  OutDataTypeStr=boolean
  Product : Product
  Sum : Sum
  Switch1 : Switch  SaturateOnIntegerOverflow=off  InputSameDT=off
  w : Outport
  wires:
  Switch1/1 -> w/1
  Product/1 -> Gain1/1, Gain/1
  Gain1/1 -> Integrator Limited/1
  Integrator Limited/2 -> Compare To Constant2/1, Switch1/2
  Compare To Constant2/1 -> Memory1/1
  OR2/1 -> Integrator Limited/2, NOT/1
  Constant2/1 -> Switch1/3
  Memory1/1 -> OR2/1
  Reset/1 -> OR2/2
  Gain/1 -> Sum/1
  Integrator Limited/1 -> Sum/2
  Sum/1 -> Switch1/1
  in/1 -> Product/1
  NOT/1 -> Product/2
